simulink model "sim_quadrotor_16b"  (R2016b)
settings: Solver=ode4  StartTime=0.0  StopTime=25  FixedStep=0.0001  RelTol=1e-3
values from neighbouring files (symbols this model uses):
  Par_actuator = mdl_actuator_dynamics_par()    [sim_quadrotor_16b_init.m]
  Par_mdlQuad = mdl_quadrotor_par()    [sim_quadrotor_16b_init.m]    (also in sim_quadrotor_init.m)
undefined symbols (not defined in the file or in its folder): Ag_phi_rad, Ag_theta_rad, AgVel_p_radPerScnd, AgVel_q_radPerScnd, Pos_z_mtr, V_u_mtrPerScnd, V_v_mtrPerScnd, V_w_mtrPerScnd
settings Model: Creator=Nu  LastModifiedBy=Nu

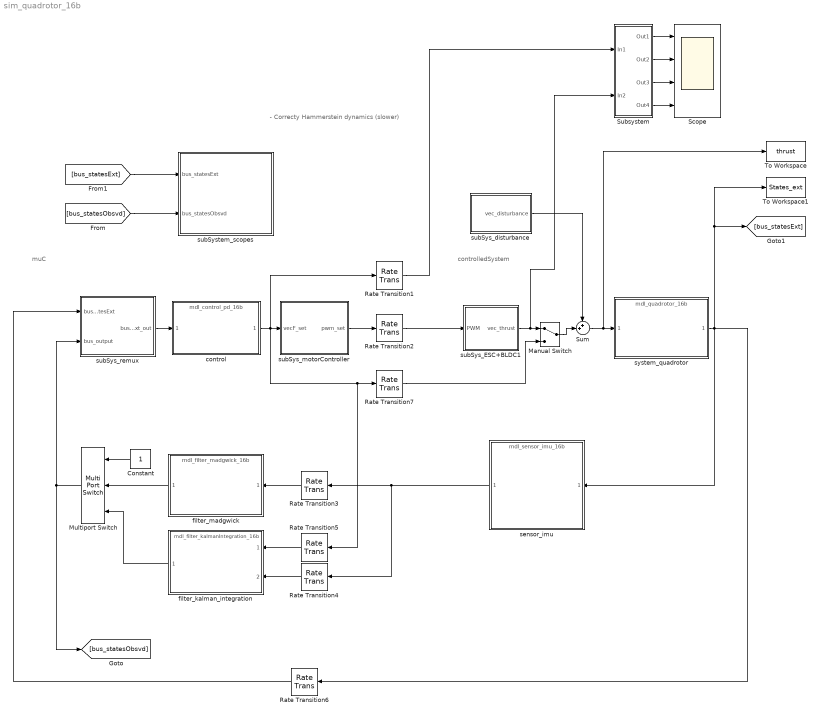
== system sim_quadrotor_16b ==
  note: - Correcty Hammerstein dynamics (slower)
  note: controlledSystem
  note: muC
  Constant : Constant
  Manual Switch : ManualSwitch
  Multiport Switch : MultiPortSwitch  DataPortOrder=Zero-based contiguous  Inputs=2
  Rate Transition{1..2,6..7} (4 alike) : RateTransition
  Rate Transition3 : RateTransition  OutPortSampleTime=Par_filterMadgwick.T
  Rate Transition4 : RateTransition  OutPortSampleTime=Par_filterKalman.T
  Rate Transition5 : RateTransition  X0=Par_mdlQuad.F0*ones(4,1)
  Scope : Scope  NumInputPorts=4
  Subsystem : Subsystem
  Sum : Sum  Inputs=++|
  To Workspace : ToWorkspace  VariableName=thrust  SaveFormat=Timeseries  SampleTime=-1
  To Workspace1 : ToWorkspace  VariableName=States_ext  SaveFormat=Timeseries  SampleTime=-1
  control : ModelReference  ModelNameDialog=mdl_control_pd_16b.slx  SimulationMode=Normal  ModelReferenceVersion=1.281
  filter_kalman_integration : ModelReference  ModelNameDialog=mdl_filter_kalmanIntegration_16b.slx  SimulationMode=Normal  ModelReferenceVersion=1.174
  filter_madgwick : ModelReference  ModelNameDialog=mdl_filter_madgwick_16b.slx  SimulationMode=Normal  ModelReferenceVersion=1.85
  sensor_imu : ModelReference  ModelNameDialog=mdl_sensor_imu_16b.slx  SimulationMode=Normal  ModelReferenceVersion=1.283
  subSys_ESC+BLDC1 : Subsystem
  subSys_disturbance : Subsystem
  subSys_motorController : Subsystem
  subSys_remux : Subsystem
  subSystem_scopes : Subsystem
  system_quadrotor : ModelReference  ModelNameDialog=mdl_quadrotor_16b.slx  SimulationMode=Normal  ModelReferenceVersion=1.338
  wires:
  sensor_imu/1 -> Rate Transition3/1, Rate Transition4/1
  [bus_statesObsvd] -> subSystem_scopes/2(bus_statesObsvd)
  [bus_statesExt] -> subSystem_scopes/1(bus_statesExt)
  Rate Transition2/1 -> subSys_ESC+BLDC1/1(PWM)
  Multiport Switch/1 -> [bus_statesObsvd], subSys_remux/2(bus_output)
  Rate Transition3/1 -> filter_madgwick/1
  filter_kalman_integration/1 -> Multiport Switch/3
  filter_madgwick/1 -> Multiport Switch/2
  Constant/1 -> Multiport Switch/1
  Rate Transition4/1 -> filter_kalman_integration/2
  system_quadrotor/1 -> To Workspace1/1, [bus_statesExt], Rate Transition6/1, sensor_imu/1
  subSys_remux/1(bus_statesExt_out) -> control/1
  Rate Transition5/1 -> filter_kalman_integration/1
  subSys_motorController/1(pwm_set) -> Rate Transition2/1
  subSys_disturbance/1(vec_disturbance) -> Sum/1
  Sum/1 -> To Workspace/1, system_quadrotor/1
  Manual Switch/1 -> Sum/2
  control/1 -> Rate Transition1/1, Rate Transition7/1, Rate Transition5/1, subSys_motorController/1(vecF_set)
  Rate Transition7/1 -> Manual Switch/2
  Rate Transition6/1 -> subSys_remux/1(bus_statesExt)
  subSys_ESC+BLDC1/1(vec_thrust) -> Subsystem/2(In2), Manual Switch/1
  Rate Transition1/1 -> Subsystem/1(In1)
  Subsystem/1(Out1) -> Scope/1
  Subsystem/2(Out2) -> Scope/2
  Subsystem/3(Out3) -> Scope/3
  Subsystem/4(Out4) -> Scope/4

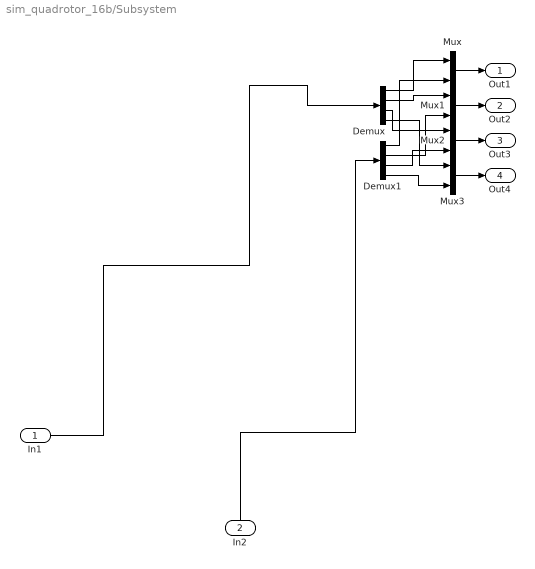
== system sim_quadrotor_16b/Subsystem ==
  In1 : Inport
  In2 : Inport  Port=2
  Demux : Demux
  Demux1 : Demux
  Mux{,1..3} (4 alike) : Mux  Inputs=2
  Out1 : Outport
  Out2 : Outport  Port=2
  Out3 : Outport  Port=3
  Out4 : Outport  Port=4
  wires:
  Demux/2 -> Mux1/1
  Mux/1 -> Out1/1
  Demux/1 -> Mux/1
  Mux2/1 -> Out3/1
  In1/1 -> Demux/1
  In2/1 -> Demux1/1
  Demux1/4 -> Mux3/2
  Demux1/2 -> Mux1/2
  Mux3/1 -> Out4/1
  Demux1/1 -> Mux/2
  Mux1/1 -> Out2/1
  Demux/3 -> Mux2/1
  Demux1/3 -> Mux2/2
  Demux/4 -> Mux3/1

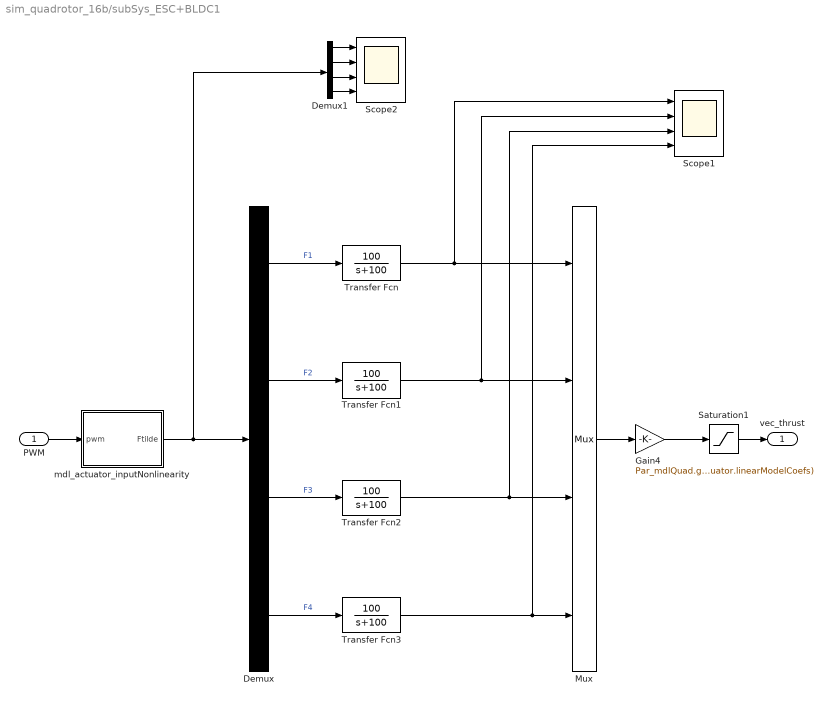
== system sim_quadrotor_16b/subSys_ESC+BLDC1 ==
  PWM : Inport
  Demux : Demux
  Demux1 : Demux
  Gain4 : Gain  Gain=Par_mdlQuad.g/sum(Par_actuator.linearModelCoefs)
  Mux : Mux
  Saturation1 : Saturate  UpperLimit=inf  LowerLimit=-inf
  Scope1 : Scope  NumInputPorts=4
  Scope2 : Scope  NumInputPorts=4
  Transfer Fcn{,1..3} (4 alike) : TransferFcn  Numerator=[100]  Denominator=[1 100]
  mdl_actuator_inputNonlinearity : MATLAB Function  TreatAsAtomicUnit=on
  vec_thrust : Outport
  wires:
  Transfer Fcn3/1 -> Mux/4, Scope1/4
  Mux/1 -> Gain4/1
  PWM/1 -> mdl_actuator_inputNonlinearity/1(pwm)
  Demux/3 -> Transfer Fcn2/1  "F3"
  Demux/4 -> Transfer Fcn3/1  "F4"
  Demux/2 -> Transfer Fcn1/1  "F2"
  Demux/1 -> Transfer Fcn/1  "F1"
  mdl_actuator_inputNonlinearity/1(Ftilde) -> Demux1/1, Demux/1
  Transfer Fcn/1 -> Mux/1, Scope1/1
  Transfer Fcn1/1 -> Mux/2, Scope1/2
  Transfer Fcn2/1 -> Mux/3, Scope1/3
  Saturation1/1 -> vec_thrust/1
  Demux1/1 -> Scope2/1
  Demux1/2 -> Scope2/2
  Demux1/3 -> Scope2/3
  Demux1/4 -> Scope2/4
  Gain4/1 -> Saturation1/1

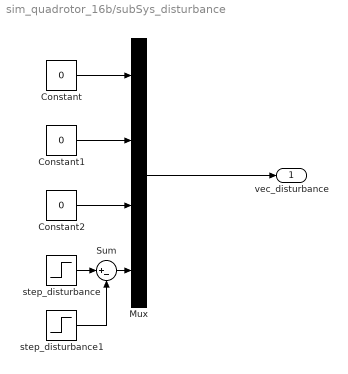
== system sim_quadrotor_16b/subSys_disturbance ==
  Constant : Constant  Value=0
  Constant1 : Constant  Value=0
  Constant2 : Constant  Value=0
  Mux : Mux
  Sum : Sum  Inputs=|+-
  step_disturbance : Step  Time=10  After=0.1  SampleTime=0
  step_disturbance1 : Step  Time=10.5  After=0.1  SampleTime=0
  vec_disturbance : Outport
  wires:
  Sum/1 -> Mux/4
  Constant/1 -> Mux/1
  Constant1/1 -> Mux/2
  Constant2/1 -> Mux/3
  step_disturbance1/1 -> Sum/2
  step_disturbance/1 -> Sum/1
  Mux/1 -> vec_disturbance/1

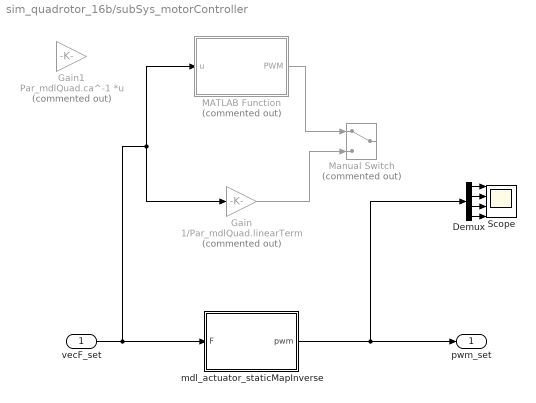
== system sim_quadrotor_16b/subSys_motorController ==
  vecF_set : Inport
  Demux : Demux
  Gain : Gain  Commented=on  Gain=1/Par_mdlQuad.linearTerm
  Gain1 : Gain  Commented=on  Gain=Par_mdlQuad.ca^-1  Multiplication=Matrix(K*u)
  MATLAB Function : MATLAB Function  Commented=on  TreatAsAtomicUnit=on
  Manual Switch : ManualSwitch  Commented=on
  Scope : Scope  NumInputPorts=4
  mdl_actuator_staticMapInverse : MATLAB Function  TreatAsAtomicUnit=on
  pwm_set : Outport
  wires:
  vecF_set/1 -> Gain/1, MATLAB Function/1(u), mdl_actuator_staticMapInverse/1(F)
  MATLAB Function/1(PWM) -> Manual Switch/1
  Gain/1 -> Manual Switch/2
  mdl_actuator_staticMapInverse/1(pwm) -> Demux/1, pwm_set/1
  Demux/1 -> Scope/1
  Demux/2 -> Scope/2
  Demux/3 -> Scope/3
  Demux/4 -> Scope/4

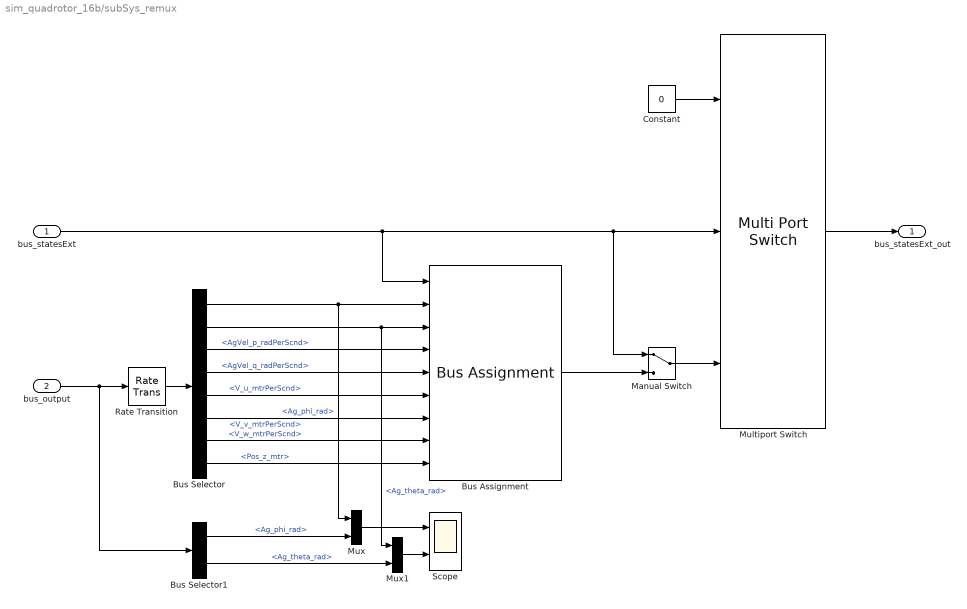
== system sim_quadrotor_16b/subSys_remux ==
  bus_statesExt : Inport
  bus_output : Inport  Port=2
  Bus Assignment : BusAssignment  AssignedSignals=Ag_phi_rad,Ag_theta_rad,AgVel_p_radPerScnd,AgVel_q_radPerScnd,V_u_mtrPerScnd,V_v_mtrPerScnd,V_w_mtrPerScnd,Pos_z_mtr
  Bus Selector : BusSelector  OutputSignals=Ag_phi_rad,Ag_theta_rad,AgVel_p_radPerScnd,AgVel_q_radPerScnd,V_u_mtrPerScnd,V_v_mtrPerScnd,V_w_mtrPerScnd,Pos_z_mtr
  Bus Selector1 : BusSelector  OutputSignals=Ag_phi_rad,Ag_theta_rad
  Constant : Constant  Value=0
  Manual Switch : ManualSwitch
  Multiport Switch : MultiPortSwitch  DataPortOrder=Zero-based contiguous  Inputs=2
  Mux : Mux  Inputs=2
  Mux1 : Mux  Inputs=2
  Rate Transition : RateTransition
  Scope : Scope  NumInputPorts=2
  bus_statesExt_out : Outport
  wires:
  Bus Selector/2 -> Mux1/1, Bus Assignment/3  "<Ag_theta_rad>"
  Bus Selector/1 -> Mux/1, Bus Assignment/2  "<Ag_phi_rad>"
  Multiport Switch/1 -> bus_statesExt_out/1
  Constant/1 -> Multiport Switch/1
  bus_statesExt/1 -> Manual Switch/1, Multiport Switch/2, Bus Assignment/1
  bus_output/1 -> Rate Transition/1, Bus Selector1/1
  Bus Assignment/1 -> Manual Switch/2
  Rate Transition/1 -> Bus Selector/1
  Bus Selector1/1 -> Mux/2  "<Ag_phi_rad>"
  Mux/1 -> Scope/1
  Mux1/1 -> Scope/2
  Bus Selector1/2 -> Mux1/2  "<Ag_theta_rad>"
  Bus Selector/3 -> Bus Assignment/4  "<AgVel_p_radPerScnd>"
  Bus Selector/4 -> Bus Assignment/5  "<AgVel_q_radPerScnd>"
  Bus Selector/5 -> Bus Assignment/6  "<V_u_mtrPerScnd>"
  Bus Selector/6 -> Bus Assignment/7  "<V_v_mtrPerScnd>"
  Manual Switch/1 -> Multiport Switch/3
  Bus Selector/7 -> Bus Assignment/8  "<V_w_mtrPerScnd>"
  Bus Selector/8 -> Bus Assignment/9  "<Pos_z_mtr>"

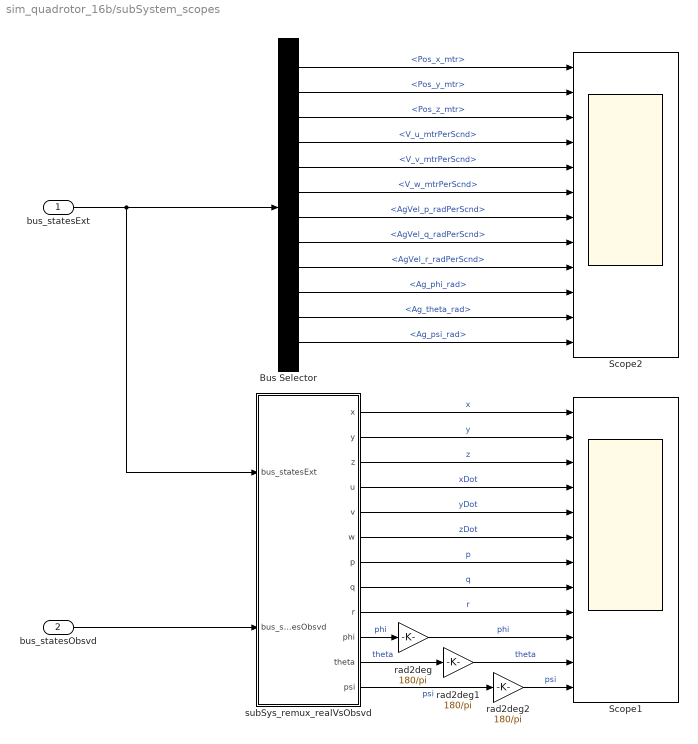
== system sim_quadrotor_16b/subSystem_scopes ==
  bus_statesExt : Inport
  bus_statesObsvd : Inport  Port=2
  Bus Selector : BusSelector  OutputSignals=Pos_x_mtr,Pos_y_mtr,Pos_z_mtr,V_u_mtrPerScnd,V_v_mtrPerScnd,V_w_mtrPerScnd,AgVel_p_radPerScnd,AgVel_q_radPerScnd,AgVel_r_radPerScnd,Ag_phi_rad,Ag_theta_rad,Ag_psi_rad
  Scope1 : Scope  NumInputPorts=12
  Scope2 : Scope  NumInputPorts=12
  rad2deg : Gain  Gain=180/pi
  rad2deg1 : Gain  Gain=180/pi
  rad2deg2 : Gain  Gain=180/pi
  subSys_remux_realVsObsvd : Subsystem
  wires:
  subSys_remux_realVsObsvd/1(x) -> Scope1/1  "x"
  subSys_remux_realVsObsvd/2(y) -> Scope1/2  "y"
  subSys_remux_realVsObsvd/3(z) -> Scope1/3  "z"
  subSys_remux_realVsObsvd/7(p) -> Scope1/7  "p"
  subSys_remux_realVsObsvd/8(q) -> Scope1/8  "q"
  subSys_remux_realVsObsvd/9(r) -> Scope1/9  "r"
  subSys_remux_realVsObsvd/10(phi) -> rad2deg/1  "phi"
  subSys_remux_realVsObsvd/11(theta) -> rad2deg1/1  "theta"
  subSys_remux_realVsObsvd/12(psi) -> rad2deg2/1  "psi"
  bus_statesExt/1 -> Bus Selector/1, subSys_remux_realVsObsvd/1(bus_statesExt)
  bus_statesObsvd/1 -> subSys_remux_realVsObsvd/2(bus_statesObsvd)
  rad2deg/1 -> Scope1/10  "phi"
  rad2deg1/1 -> Scope1/11  "theta"
  rad2deg2/1 -> Scope1/12  "psi"
  Bus Selector/1 -> Scope2/1  "<Pos_x_mtr>"
  Bus Selector/2 -> Scope2/2  "<Pos_y_mtr>"
  Bus Selector/3 -> Scope2/3  "<Pos_z_mtr>"
  Bus Selector/4 -> Scope2/4  "<V_u_mtrPerScnd>"
  Bus Selector/5 -> Scope2/5  "<V_v_mtrPerScnd>"
  Bus Selector/6 -> Scope2/6  "<V_w_mtrPerScnd>"
  Bus Selector/7 -> Scope2/7  "<AgVel_p_radPerScnd>"
  Bus Selector/8 -> Scope2/8  "<AgVel_q_radPerScnd>"
  Bus Selector/9 -> Scope2/9  "<AgVel_r_radPerScnd>"
  Bus Selector/10 -> Scope2/10  "<Ag_phi_rad>"
  Bus Selector/11 -> Scope2/11  "<Ag_theta_rad>"
  Bus Selector/12 -> Scope2/12  "<Ag_psi_rad>"
  subSys_remux_realVsObsvd/4(u) -> Scope1/4  "xDot"
  subSys_remux_realVsObsvd/5(v) -> Scope1/5  "yDot"
  subSys_remux_realVsObsvd/6(w) -> Scope1/6  "zDot"

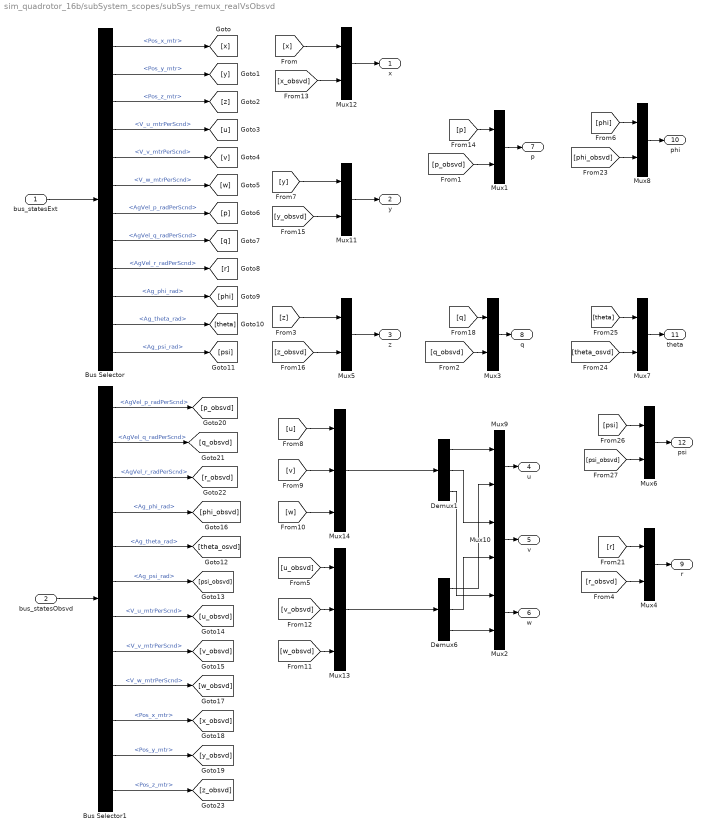
== system sim_quadrotor_16b/subSystem_scopes/subSys_remux_realVsObsvd ==
  bus_statesExt : Inport
  bus_statesObsvd : Inport  Port=2
  Bus Selector : BusSelector  OutputSignals=Pos_x_mtr,Pos_y_mtr,Pos_z_mtr,V_u_mtrPerScnd,V_v_mtrPerScnd,V_w_mtrPerScnd,AgVel_p_radPerScnd,AgVel_q_radPerScnd,AgVel_r_radPerScnd,Ag_phi_rad,Ag_theta_rad,Ag_psi_rad
  Bus Selector1 : BusSelector  OutputSignals=AgVel_p_radPerScnd,AgVel_q_radPerScnd,AgVel_r_radPerScnd,Ag_phi_rad,Ag_theta_rad,Ag_psi_rad,V_u_mtrPerScnd,V_v_mtrPerScnd,V_w_mtrPerScnd,Pos_x_mtr,Pos_y_mtr,Pos_z_mtr
  Demux1 : Demux  Outputs=3
  Demux6 : Demux  Outputs=3
  Mux{1..12} (12 alike) : Mux  Inputs=2
  Mux13 : Mux  Inputs=3
  Mux14 : Mux  Inputs=3
  x : Outport
  y : Outport  Port=2
  z : Outport  Port=3
  u : Outport  Port=4
  v : Outport  Port=5
  w : Outport  Port=6
  p : Outport  Port=7
  q : Outport  Port=8
  r : Outport  Port=9
  phi : Outport  Port=10
  theta : Outport  Port=11
  psi : Outport  Port=12
  wires:
  [z] -> Mux5/1
  [z_obsvd] -> Mux5/2
  Bus Selector1/3 -> [r_obsvd]  "<AgVel_r_radPerScnd>"
  Bus Selector1/2 -> [q_obsvd]  "<AgVel_q_radPerScnd>"
  Bus Selector1/1 -> [p_obsvd]  "<AgVel_p_radPerScnd>"
  Bus Selector/9 -> [r]  "<AgVel_r_radPerScnd>"
  Bus Selector/10 -> [phi]  "<Ag_phi_rad>"
  Bus Selector/11 -> [theta]  "<Ag_theta_rad>"
  Bus Selector/12 -> [psi]  "<Ag_psi_rad>"
  Bus Selector/8 -> [q]  "<AgVel_q_radPerScnd>"
  Bus Selector/7 -> [p]  "<AgVel_p_radPerScnd>"
  Bus Selector/6 -> [w]  "<V_w_mtrPerScnd>"
  Bus Selector/5 -> [v]  "<V_v_mtrPerScnd>"
  Bus Selector/4 -> [u]  "<V_u_mtrPerScnd>"
  Bus Selector/2 -> [y]  "<Pos_y_mtr>"
  Bus Selector/3 -> [z]  "<Pos_z_mtr>"
  Mux2/1 -> w/1
  Mux5/1 -> z/1
  bus_statesObsvd/1 -> Bus Selector1/1
  bus_statesExt/1 -> Bus Selector/1
  Bus Selector/1 -> [x]  "<Pos_x_mtr>"
  [w] -> Mux14/3
  [w_obsvd] -> Mux13/3
  [p] -> Mux1/1
  [p_obsvd] -> Mux1/2
  [q] -> Mux3/1
  [q_obsvd] -> Mux3/2
  [r] -> Mux4/1
  [r_obsvd] -> Mux4/2
  [psi] -> Mux6/1
  [psi_obsvd] -> Mux6/2
  [theta] -> Mux7/1
  [theta_osvd] -> Mux7/2
  [phi] -> Mux8/1
  [phi_obsvd] -> Mux8/2
  Mux1/1 -> p/1
  Mux3/1 -> q/1
  Mux4/1 -> r/1
  Mux6/1 -> psi/1
  Mux7/1 -> theta/1
  Mux8/1 -> phi/1
  Bus Selector1/5 -> [theta_osvd]  "<Ag_theta_rad>"
  Bus Selector1/6 -> [psi_obsvd]  "<Ag_psi_rad>"
  Bus Selector1/4 -> [phi_obsvd]  "<Ag_phi_rad>"
  Bus Selector1/7 -> [u_obsvd]  "<V_u_mtrPerScnd>"
  Bus Selector1/8 -> [v_obsvd]  "<V_v_mtrPerScnd>"
  Bus Selector1/9 -> [w_obsvd]  "<V_w_mtrPerScnd>"
  Mux9/1 -> u/1
  [u] -> Mux14/1
  [u_obsvd] -> Mux13/1
  Mux10/1 -> v/1
  [v] -> Mux14/2
  [v_obsvd] -> Mux13/2
  Bus Selector1/12 -> [z_obsvd]  "<Pos_z_mtr>"
  Bus Selector1/11 -> [y_obsvd]  "<Pos_y_mtr>"
  Bus Selector1/10 -> [x_obsvd]  "<Pos_x_mtr>"
  [y_obsvd] -> Mux11/2
  [y] -> Mux11/1
  Mux11/1 -> y/1
  [x_obsvd] -> Mux12/2
  [x] -> Mux12/1
  Mux12/1 -> x/1
  Mux13/1 -> Demux6/1
  Mux14/1 -> Demux1/1
  Demux1/1 -> Mux9/1
  Demux6/1 -> Mux9/2
  Demux1/2 -> Mux10/1
  Demux6/2 -> Mux10/2
  Demux1/3 -> Mux2/1
  Demux6/3 -> Mux2/2

== matlab function sim_quadrotor_16b/subSys_motorController/mdl_actuator_staticMapInverse ==
  data: F input; pwm output
function pwm = fcn( F )

pwm = mdl_actuator_staticMapInverse( F );

== matlab function sim_quadrotor_16b/subSys_ESC+BLDC1/mdl_actuator_inputNonlinearity ==
  data: pwm input; Ftilde output
function Ftilde = fcn( pwm )

Ftilde = mdl_actuator_inputNonlinearity( pwm );

== matlab function sim_quadrotor_16b/subSys_motorController/MATLAB Function ==
  data: u input; PWM output; Par_mdlQuad parameter
function PWM = fcn(u, Par_mdlQuad)

% pwm = Par_mdlQuad.ca_esc^-1 * u;
pwm = u/Par_mdlQuad.linearTerm;
PWM = pwm + Par_mdlQuad.PWM0;
